simulink model "pos_control_tracking"  (R2022b)
settings: Solver=VariableStepAuto  StartTime=0.0  StopTime=2  RelTol=1e-3
values from neighbouring files (symbols this model uses):
  lbu_leg = repmat(leg_model_obj.input_constraints(:,1),Nl,1)    [initialize_sim_parameters.m]    (also in pos_control_setup.m)
  lbx_leg = repmat(leg_model_obj.state_constraints(:,1),Nl-1,1)    [initialize_sim_parameters.m]    (also in pos_control_setup.m)
  lg_leg = repmat(lower_g,Nl,1)    [initialize_sim_parameters.m]    (also in pos_control_setup.m)
  lh_leg = repmat([0;0],Nl,1)    [initialize_sim_parameters.m]    (also in pos_control_setup.m)
  Nl = 40    [initialize_sim_parameters.m]    (also in pos_control_setup.m = 30)
  nu = 3    [pos_control_setup.m]    (also in traj_player_prepar.m)
  nu_l = 3    [initialize_sim_parameters.m]    (also in pos_control_setup.m)
  nx = 10    [pos_control_setup.m]    (also in traj_player_prepar.m)
  nx_l = 10    [initialize_sim_parameters.m]    (also in pos_control_setup.m)
  Th = 1.5    [pos_control_setup.m]    (also in traj_player_prepar.m = 0.75)
  ubu_leg = repmat(leg_model_obj.input_constraints(:,2),Nl,1)    [initialize_sim_parameters.m]    (also in pos_control_setup.m)
  ubx_leg = repmat(leg_model_obj.state_constraints(:,2),Nl-1,1)    [initialize_sim_parameters.m]    (also in pos_control_setup.m)
  ug_leg = repmat(upper_g,Nl,1)    [initialize_sim_parameters.m]    (also in pos_control_setup.m)
  uh_leg = repmat([0;0],Nl,1)    [initialize_sim_parameters.m]    (also in pos_control_setup.m)
  y_ref_sim = repmat(y_ref,N-1,1)    [pos_control_setup.m]
libraries: simulink x2, sm_lib x2, slpidlib x1, nesl_utility x1
settings Model: Creator=papaveneti  LastModifiedBy=papaveneti

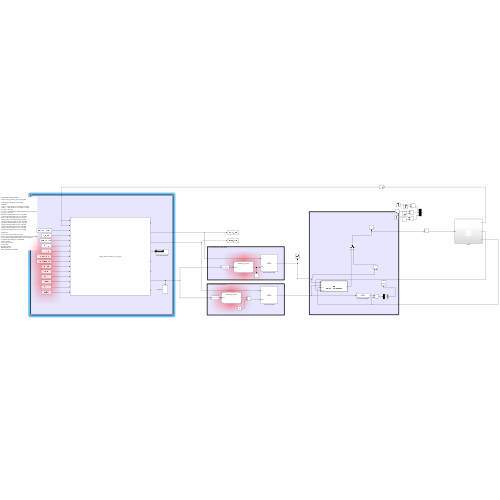
[thumbnail: Simulink's stored preview of the top-level diagram]
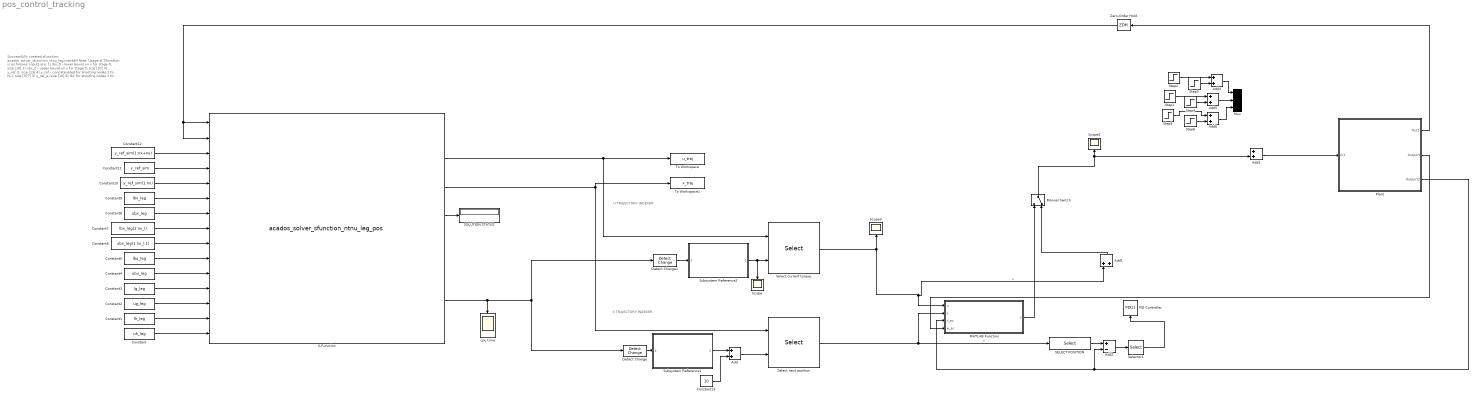
== system pos_control_tracking ==
  note: U TRAJECTORY INDEXER
  note: X TRAJECTORY INDEXER
  note: Successfully created sfunction:
      | acados_solver_sfunction_ntnu_leg.mexa64
      |
      | Note: Usage of Sfunction is as follows:
      | Inputs are:
      | 1) lbx_0 - lower bound on x for stage 0, size [10]
      | 2) ubx_0 - upper bound on x for stage 0, size [10]
      | 3) y_ref_0, size [13]
      | 4) y_ref - concatenated for shooting nodes 1 to N-1, size [377]
      | 5) y_ref_e, size [10]
      | 6) lbx for shooting nodes 1 to N-1, size [290]
      | 7) ubx for shooting nodes 1 to N-1, size [290]
      | 8) lbx_e (lbx at shooting node N), size [10]
      | 9) ubx_e (ubx at shooting node N), size [10]
      | 10) lbu for shooting nodes 0 to N-1, size [90]
      | 11) ubu for shooting nodes 0 to N-1, size [90]
      | 12) lg for shooting nodes 0 to N-1, size [60]
      | 13) ug for shooting nodes 0 to N-1, size [60]
      | 14) lh for shooting nodes 0 to N-1, size [60]
      | 15) uh for shooting nodes 0 to N-1, size [60]
      |
      | Outputs are:
      | 1) u0, control input at node 0, size [3]
      | 2) utraj, control input concatenated for nodes 0 to N-1, size [90]
      | 3) xtraj, state concatenated for nodes 0 to N, size [310]
      | 4) acados solver status (0 = SUCCESS)
      | 5) KKT residual
      | 6) x1, state at node 1
      | 7) CPU time
      | 8) SQP iterations
      | Building with 'gcc'.
      | MEX completed successfully.
  Add{,1,3..6} (6 alike) : Sum
  Add2 : Sum  Inputs=+-
  Constant : Constant  Value=uh_leg
  Constant1 : Constant  Value=lh_leg
  Constant10 : Constant  Value=y_ref_sim(1:nx)
  Constant11 : Constant  Value=y_ref_sim
  Constant12 : Constant  Value=y_ref_sim(1:nx+nu)
  Constant13 : Constant  Value=10
  Constant2 : Constant  Value=ug_leg
  Constant3 : Constant  Value=lg_leg
  Constant4 : Constant  Value=ubu_leg
  Constant5 : Constant  Value=lbu_leg
  Constant6 : Constant  Value=ubx_leg(1:nx_l,1)
  Constant7 : Constant  Value=lbx_leg(1:nx_l)
  Constant8 : Constant  Value=ubx_leg
  Constant9 : Constant  Value=lbx_leg
  Detect Change : simulink/Logic and Bit Operations/Detect Change  vinit=0  OutDataTypeStr=boolean
  Detect Change1 : simulink/Logic and Bit Operations/Detect Change  vinit=0  OutDataTypeStr=boolean
  MATLAB Function : MATLAB Function  TreatAsAtomicUnit=on
  Manual Switch : ManualSwitch  CurrentSetting=0
  Mux : Mux  Inputs=3
  PID Controller : slpidlib/PID Controller  Controller=PD  Form=Parallel  TimeDomain=Discrete-time  UseExternalTs=off  SampleTime=1e-3  IntegratorMethod=Forward Euler  FilterMethod=Forward Euler  ControllerParametersSource=internal  P=1  I=1  UseKiTs=off  D=0.1  N=50  UseFilter=on  TunerSelectOption=Transfer Function Based (PID Tuner App)  InitialConditionSource=internal  InitialConditionForIntegrator=0  InitialConditionForFilter=0  DifferentiatorICPrevScaledInput=0  ExternalReset=none  TrackingMode=off  Kt=1  LimitOutput=off  SatLimitsSource=internal  UpperSaturationLimit=inf  LowerSaturationLimit=-inf  LinearizeAsGain=on  AntiWindupMode=none  Kb=1  LimitIntegrator=off  UpperIntegratorSaturationLimit=inf  LowerIntegratorSaturationLimit=-inf  POutMin=[]  POutMax=[]  IOutMin=[]  IOutMax=[]  DOutMin=[]  DOutMax=[]  NOutMin=[]  NOutMax=[]  SumOutMin=[]  SumOutMax=[]  SaturationOutMin=[]  SaturationOutMax=[]  PParamMin=[]  PParamMax=[]  IParamMin=[]  IParamMax=[]  DParamMin=[]  DParamMax=[]  NParamMin=[]  NParamMax=[]  KbParamMin=[]  KbParamMax=[]  KtParamMin=[]  KtParamMax=[]  KbOutMin=[]  KbOutMax=[]  KtOutMin=[]  KtOutMax=[]  IntegratorOutMin=[]  IntegratorOutMax=[]  FilterOutMin=[]  FilterOutMax=[]  SumI1OutMin=[]  SumI1OutMax=[]  SumI2OutMin=[]  SumI2OutMax=[]  SumI3OutMin=[]  SumI3OutMax=[]  SumI4OutMin=[]  SumI4OutMax=[]  SumDOutMin=[]  SumDOutMax=[]  DifferentiatorOutMin=[]  DifferentiatorOutMax=[]  FilterDiffOutCoefMin=[]  FilterDiffOutCoefMax=[]  ReciprocalOutMin=[]  ReciprocalOutMax=[]  SumDenOutMin=[]  SumDenOutMax=[]  SumNumOutMin=[]  SumNumOutMax=[]  DivideOutMin=[]  DivideOutMax=[]  UdiffTsProdOutMin=[]  UdiffTsProdOutMax=[]  NTsProdOutMin=[]  NTsProdOutMax=[]  UintegralTsProdOutMin=[]  UintegralTsProdOutMax=[]  UngainTsProdOutMin=[]  UngainTsProdOutMax=[]  ClampingZeroOutDataTypeStr=Inherit: Inherit via back propagation  ClampingZeroOutMin=[]  ClampingZeroOutMax=[]  FilterDenConstantOutDataTypeStr=Inherit: Inherit via back propagation  FilterDenConstantOutMin=[]  FilterDenConstantOutMax=[]  PCopyOutDataTypeStr=Inherit: Inherit via back propagation  PCopyOutMin=[]  PCopyOutMax=[]  NCopyOutDataTypeStr=Inherit: Inherit via back propagation  NCopyOutMin=[]  NCopyOutMax=[]  IntegratorContinuousStateAttributes=''  IntegratorStateMustResolveToSignalObject=off  IntegratorRTWStateStorageClass=Auto  FilterContinuousStateAttributes=''  FilterStateMustResolveToSignalObject=off  FilterRTWStateStorageClass=Auto  ParallelPVariant=InternalParameters  IdealPVariant=Disabled  IVariant=Disabled  DVariant=InternalParameters  IntegratorVariant=Disabled  SatVariant=Disabled  AWVariant=Disabled  PCopyVariant=Disabled  TRVariant=Disabled  FdbkBlocksVariant=Forward  IdealPFdbkVariant=Disabled  SatFdbkVariant=Disabled  DerivativeFilterVariant=ForwardEulerFilter  NVariant=InternalParameters  NCopyVariant=Disabled  FilterICVariant=InternalICsFilter  IntegratorICVariant=Disabled  ExternalResetVariant=Disabled  TRSumVariant=Passthrough  SumFdbkVariant=Disabled  SumVariant=Sum_PD  TsampFilterVariant=InternalTs  TsampNgainVariant=Passthrough  TsampIntegralVariant=Disabled_SignalSpec  ExternalSaturationOutDataTypeStr=Inherit: Same as second input
  Plant : Subsystem
  S-Function : S-Function  FunctionName=acados_solver_sfunction_ntnu_leg_pos  SFunctionDeploymentMode=off  EnableBusSupport=off
  SELECT POSITION : Selector  InputPortWidth=10  IndexOptions=Index vector (dialog)  Indices=[1,2,3,4,5]  OutputSizes=1
  SOLUTION STATUS : Display
  Scope : Scope
  Scope2 : Scope
  Scope3 : Scope
  Select current torque : Selector  InputPortWidth=90  IndexOptions=Starting index (port)  Indices=[1 3]  OutputSizes=3
  Select next position : Selector  InputPortWidth=310  IndexOptions=Starting index (port)  Indices=[1 3]  OutputSizes=10
  Selector1 : Selector  InputPortWidth=5  IndexOptions=Index vector (dialog)  Indices=[1,2,4]  OutputSizes=1
  Step1 : Step  Time=0.3  After=2.5  SampleTime=0
  Step2 : Step  Time=0.5  After=-3  SampleTime=0
  Step3 : Step  Time=0.52  After=+3  SampleTime=0
  Step4 : Step  Time=0.32  After=-2.5  SampleTime=0
  Step5 : Step  Time=0.6  After=-2.5  SampleTime=0
  Step6 : Step  Time=0.62  After=2.5  SampleTime=0
  Subsystem Reference1 : Subsystem  ReferencedSubsystem=overflowing_counter  Td=Th/Nl  Overflow_point=(Nl)*nx_l  Increment=nx_l
  Subsystem Reference2 : Subsystem  ReferencedSubsystem=overflowing_counter  Td=Th/Nl  Overflow_point=(Nl)*nu_l  Increment=nu_l
  To Workspace : ToWorkspace  VariableName=u_traj  SaveFormat=Timeseries  SampleTime=-1
  To Workspace1 : ToWorkspace  VariableName=x_traj  SaveFormat=Timeseries  SampleTime=-1
  Zero-Order Hold : ZeroOrderHold  SampleTime=1.5
  cpu time : Scope
  wires:
  Zero-Order Hold/1 -> S-Function/2, S-Function/1
  Constant/1 -> S-Function/15
  Constant1/1 -> S-Function/14
  Constant2/1 -> S-Function/13
  Constant3/1 -> S-Function/12
  Constant4/1 -> S-Function/11
  Constant5/1 -> S-Function/10
  Constant6/1 -> S-Function/9
  Constant7/1 -> S-Function/8
  Constant8/1 -> S-Function/7
  Constant9/1 -> S-Function/6
  Constant10/1 -> S-Function/5
  Constant11/1 -> S-Function/4
  Constant12/1 -> S-Function/3
  S-Function/3 -> To Workspace1/1, Select next position/1
  Detect Change/1 -> Subsystem Reference1/1
  Detect Change1/1 -> Subsystem Reference2/1
  Subsystem Reference2/1 -> Select current torque/2, Scope/1
  S-Function/2 -> To Workspace/1, Select current torque/1
  Add/1 -> Select next position/2
  Subsystem Reference1/1 -> Add/1
  Constant13/1 -> Add/2
  Select current torque/1 -> Add1/1, MATLAB Function/1(u), Scope3/1  "u"
  Select next position/1 -> MATLAB Function/2(x), SELECT POSITION/1  "x"
  S-Function/4 -> SOLUTION STATUS/1
  MATLAB Function/1(y) -> Manual Switch/1
  Manual Switch/1 -> Scope2/1, Add3/2
  Add2/1 -> Selector1/1
  Selector1/1 -> PID Controller/1
  Add1/1 -> Manual Switch/2
  SELECT POSITION/1 -> Add2/1
  Plant/3(Outport2) -> MATLAB Function/3(x_ac), Add2/2
  Plant/1(Out1) -> Zero-Order Hold/1
  Plant/2(Outport) -> MATLAB Function/4(w_ac)
  S-Function/7 -> Detect Change/1, Detect Change1/1, cpu time/1
  Add3/1 -> Plant/1(In1)
  Step2/1 -> Add4/1
  Add4/1 -> Mux/1
  Step3/1 -> Add4/2
  Step4/1 -> Add5/2
  Step1/1 -> Add5/1
  Step5/1 -> Add6/1
  Step6/1 -> Add6/2
  Add5/1 -> Mux/2
  Add6/1 -> Mux/3

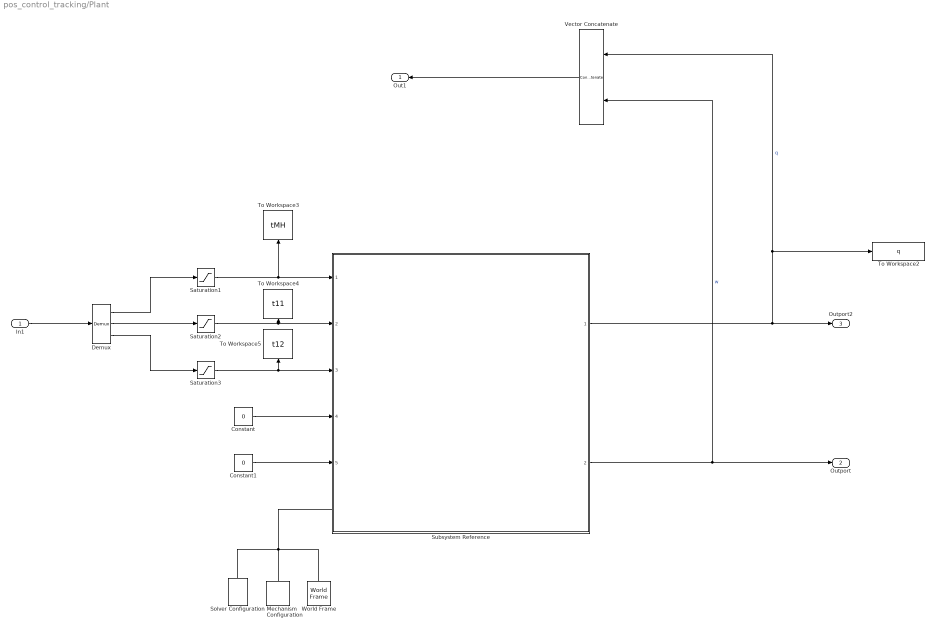
== system pos_control_tracking/Plant ==
  In1 : Inport
  Constant : Constant  Value=0
  Constant1 : Constant  Value=0
  Demux : Demux  Outputs=3
  Mechanism Configuration : sm_lib/Utilities/Mechanism Configuration  UniformGravity=Constant  GravityVector=gravity  GravityUnits=m/s^2  LinearizationDelta=0.001  JointModeTransitionNonlinearIterations=2
  Saturation1 : Saturate  UpperLimit=10  LowerLimit=-10
  Saturation2 : Saturate  UpperLimit=10  LowerLimit=-10
  Saturation3 : Saturate  UpperLimit=10  LowerLimit=-10
  Solver Configuration : nesl_utility/Solver Configuration  PhysicalDomain=network_engine_domain  SubClassName=solver  LeftPortType=input  RightPortType=generic  Tones=[]  Harmonics=[]  SimulateNoise=off  Profile=off  UseLocalSampling=off  EnableSwitchedLinearOptims=on  FrequencyDomain=off  UseCCode=off  RelTol=0.001  AbsTol=0.001  MinStep=1e-09  ToWorkspace=off  RevertToSquareIcSolve=off  NumHomotopyIterations=100  PhasorMode=off  PhasorModeNumHarmonics=1  ConsistencySolver=NEWTON_XTOL_AFTER_FTOL  IndexReductionMethod=DerivativeReplacement  DoDC=off  ResidualTolerance=1e-09  ConsistencyTolSource=GLOBAL  ConsistencyAbsTol=0.001  ConsistencyRelTol=0.001  ConsistencyTolFactor=0.001  UseLocalSolver=off  LocalSolverChoice=NE_BACKWARD_EULER_ADVANCER  ResolveIndetEquations=on  FunctionEvalNumThread=1  LocalSolverSampleTime=0.001  DoFixedCost=off  MaxNonlinIter=3  MaxModeIter=2  ComputeImpulses=off  ImpulseIterations=2  LinearAlgebra=auto  LinearAlgebraNumThread=0  EquationFormulation=NE_TIME_EF  DelaysMemoryBudget=1024  AutomaticFiltering=on  FilteringTimeConstant=0.001  PartitionStorageMethod=AS_NEEDED  PartitionMemoryBudget=1024  PartitionMethod=ROBUST
  Subsystem Reference : Subsystem  ReferencedSubsystem=ntnu_leg_torque_control
  To Workspace2 : ToWorkspace  VariableName=q  SaveFormat=Timeseries  SampleTime=-1
  To Workspace3 : ToWorkspace  VariableName=tMH  SaveFormat=Timeseries  SampleTime=-1
  To Workspace4 : ToWorkspace  VariableName=t11  SaveFormat=Timeseries  SampleTime=-1
  To Workspace5 : ToWorkspace  VariableName=t12  SaveFormat=Timeseries  SampleTime=-1
  Vector Concatenate : Concatenate
  World Frame : sm_lib/Frames and Transforms/World Frame
  Out1 : Outport
  Outport : Outport  Port=2
  Outport2 : Outport  Port=3
  wires:
  Demux/2 -> Saturation2/1
  Saturation1/1 -> Subsystem Reference/1, To Workspace3/1
  Saturation2/1 -> Subsystem Reference/2, To Workspace4/1
  In1/1 -> Demux/1
  Vector Concatenate/1 -> Out1/1
  Saturation3/1 -> Subsystem Reference/3, To Workspace5/1
  Demux/1 -> Saturation1/1
  Demux/3 -> Saturation3/1
  Subsystem Reference/2 -> Outport/1, Vector Concatenate/2  "w"
  Subsystem Reference/1 -> Vector Concatenate/1, To Workspace2/1, Outport2/1  "q"
  Constant/1 -> Subsystem Reference/4
  Constant1/1 -> Subsystem Reference/5
  connections:
  Mechanism Configuration/RConn1 -- Solver Configuration/RConn1 -- Subsystem Reference/LConn1 -- World Frame/RConn1

== matlab function pos_control_tracking/MATLAB Function ==
  data: u input; y output; x input; x_ac input; w_ac input
function y = TRACKING_CONTROLLER(u, x, x_ac, w_ac)
Kp = 10;
Kd = 5;
y = u + Kp* ( x([1,2,4])-x_ac ([1 2 4]) ) ;%+ Kd* ( x([6,7,9])-w_ac ([1 2 4]) ) ;

% y = u;
